simulink model "new_envModel_rl"  (R2020b)
settings: Solver=ode23t  StartTime=0.0  StopTime=8  RelTol=1e-2
values from neighbouring files (symbols this model uses):
  simlen = 80    [new_main_rl.m]    (also in old_main_rl.m = 5)
  Tf = simlen*Ts    [new_main_rl.m]    (also in old_main_rl.m)
  Ts = s.Ts    [new_main_rl.m]    (also in old_main_rl.m)
  ulim = s.actuatorRange    [new_main_rl.m]    (also in old_main_rl.m)
  whichAg_sim = whichAg_sim*5    (= 30)    [new_main_rl.m]    (also in old_main_rl.m)
  ylim = s.sensorRange    [new_main_rl.m]    (also in old_main_rl.m)
undefined symbols (not defined in the file or in its folder): s
libraries: rllib x3, simulink x2
settings Model: Creator=The MathWorks, Inc.  LastModifiedBy=sunan
settings DataIOCC: ExternalInput=s  SaveFormat=Structure  SaveOutput=off  SignalLogging=off  InspectSignalLogs=on  SaveTime=off  DSMLoggingName=s

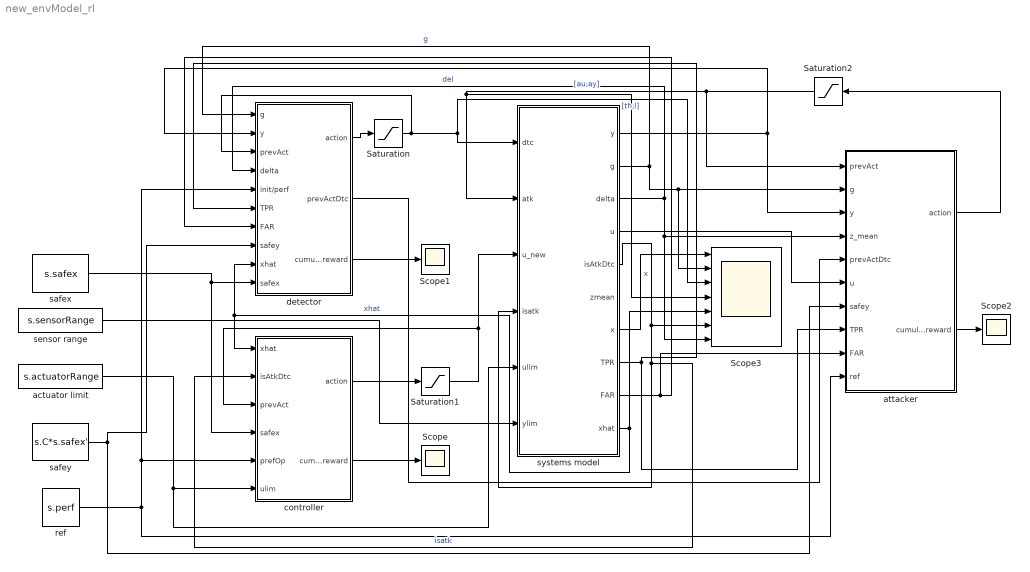
== system new_envModel_rl ==
  Saturation : Saturate  UpperLimit=[100;simlen]  LowerLimit=[0;1]
  Saturation1 : Saturate  UpperLimit=s.actuatorRange  LowerLimit=-s.actuatorRange
  Saturation2 : Saturate  UpperLimit=[ulim;ylim]  LowerLimit=-[ulim;ylim]
  Scope : Scope
  Scope1 : Scope
  Scope2 : Scope
  Scope3 : Scope  NumInputPorts=7
  actuator limit : Constant  Value=s.actuatorRange
  attacker : Subsystem
  controller : Subsystem
  detector : Subsystem
  ref : Constant  Value=s.perf
  safex : Constant  Value=s.safex
  safey : Constant  Value=s.C*s.safex'
  sensor range : Constant  Value=s.sensorRange
  systems model : Subsystem
  wires:
  systems model/1(y) -> detector/2(y), attacker/3(y)
  ref/1 -> controller/5(prefOp), detector/5(init/perf), attacker/10(ref)
  safey/1 -> attacker/7(safey), detector/8(safey)
  systems model/3(delta) -> Scope3/7, attacker/4(z_mean), detector/4(delta)  "del"
  systems model/2(g) -> detector/1(g), Scope3/2, attacker/2(g)  "g"
  sensor range/1 -> systems model/6(ylim)
  actuator limit/1 -> systems model/5(ulim), controller/6(ulim)
  Saturation/1 -> detector/3(prevAct), Scope3/3, systems model/1(dtc)  "[th;l]"
  Saturation1/1 -> systems model/3(u_new), controller/3(prevAct)
  Saturation2/1 -> attacker/1(prevAct), systems model/2(atk), Scope3/4  "[au;ay]"
  systems model/7(x) -> Scope3/1  "x"
  systems model/9(FAR) -> detector/7(FAR), attacker/9(FAR)
  systems model/8(TPR) -> attacker/8(TPR), detector/6(TPR)
  detector/1(action) -> Saturation/1
  detector/3(cumulative_reward) -> Scope1/1
  systems model/5(isAtkDtc) -> systems model/4(isatk), controller/2(isAtkDtc), Scope3/6  "isatk"
  controller/1(action) -> Saturation1/1
  controller/2(cumulative_reward) -> Scope/1
  detector/2(prevActDtc) -> attacker/5(prevActDtc)
  systems model/4(u) -> attacker/6(u)
  attacker/1(action) -> Saturation2/1
  attacker/2(cumulative_reward) -> Scope2/1
  systems model/10(xhat) -> Scope3/5, controller/1(xhat), detector/9(xhat)  "xhat"
  safex/1 -> detector/10(safex), controller/4(safex)

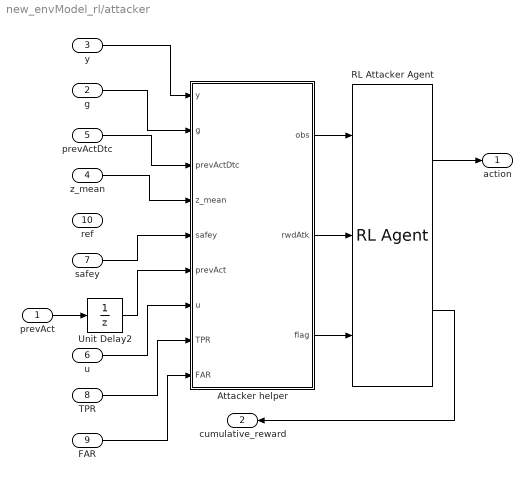
== system new_envModel_rl/attacker ==
  prevAct : Inport
  g : Inport  Port=2
  y : Inport  Port=3
  z_mean : Inport  Port=4
  prevActDtc : Inport  Port=5
  u : Inport  Port=6
  safey : Inport  Port=7
  TPR : Inport  Port=8
  FAR : Inport  Port=9
  ref : Inport  Port=10
  Attacker helper : Subsystem
  RL Attacker Agent : rllib/RL Agent  Agent=agentAtk  ProvideReward=on  ProvideIsDone=on  ProvideCumRwd=on  TreatAsDirectFeedthrough=on  CollectLoggedSignals=on  CollectModelStates=on
  Unit Delay2 : UnitDelay  SampleTime=-1  HasFrameUpgradeWarning=on
  action : Outport
  cumulative_reward : Outport  Port=2
  wires:
  z_mean/1 -> Attacker helper/4(z_mean)
  prevAct/1 -> Unit Delay2/1
  y/1 -> Attacker helper/1(y)
  Attacker helper/3(flag) -> RL Attacker Agent/3
  Attacker helper/1(obs) -> RL Attacker Agent/1
  Attacker helper/2(rwdAtk) -> RL Attacker Agent/2
  RL Attacker Agent/2 -> cumulative_reward/1
  Unit Delay2/1 -> Attacker helper/6(prevAct)
  RL Attacker Agent/1 -> action/1
  TPR/1 -> Attacker helper/8(TPR)
  FAR/1 -> Attacker helper/9(FAR)
  prevActDtc/1 -> Attacker helper/3(prevActDtc)
  g/1 -> Attacker helper/2(g)
  u/1 -> Attacker helper/7(u)
  safey/1 -> Attacker helper/5(safey)

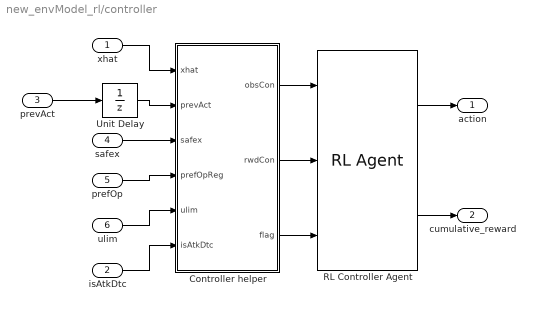
== system new_envModel_rl/controller ==
  xhat : Inport
  isAtkDtc : Inport  Port=2
  prevAct : Inport  Port=3
  safex : Inport  Port=4
  prefOp : Inport  Port=5
  ulim : Inport  Port=6
  Controller helper : Subsystem
  RL Controller Agent : rllib/RL Agent  Agent=agentCon  ProvideReward=on  ProvideIsDone=on  ProvideCumRwd=on  TreatAsDirectFeedthrough=on  CollectLoggedSignals=on  CollectModelStates=on
  Unit Delay : UnitDelay  SampleTime=-1  HasFrameUpgradeWarning=on
  action : Outport
  cumulative_reward : Outport  Port=2
  wires:
  Unit Delay/1 -> Controller helper/2(prevAct)
  RL Controller Agent/2 -> cumulative_reward/1
  prefOp/1 -> Controller helper/4(prefOpReg)
  Controller helper/1(obsCon) -> RL Controller Agent/1
  ulim/1 -> Controller helper/5(ulim)
  Controller helper/3(flag) -> RL Controller Agent/3
  safex/1 -> Controller helper/3(safex)
  prevAct/1 -> Unit Delay/1
  Controller helper/2(rwdCon) -> RL Controller Agent/2
  isAtkDtc/1 -> Controller helper/6(isAtkDtc)
  RL Controller Agent/1 -> action/1
  xhat/1 -> Controller helper/1(xhat)

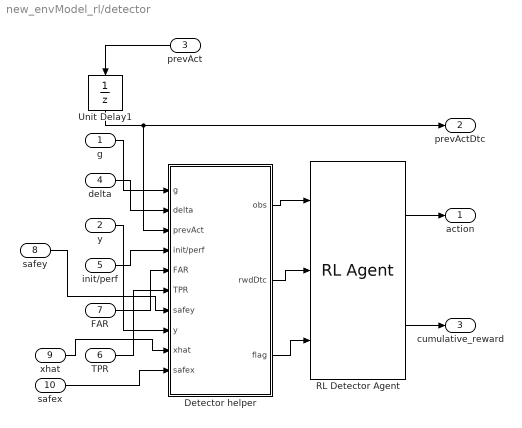
== system new_envModel_rl/detector ==
  g : Inport
  y : Inport  Port=2
  prevAct : Inport  Port=3
  delta : Inport  Port=4
  init/perf : Inport  Port=5
  TPR : Inport  Port=6
  FAR : Inport  Port=7
  safey : Inport  Port=8
  xhat : Inport  Port=9
  safex : Inport  Port=10
  Detector helper : Subsystem
  RL Detector Agent : rllib/RL Agent  Agent=agentDtc  ProvideReward=on  ProvideIsDone=on  ProvideCumRwd=on  TreatAsDirectFeedthrough=on  CollectLoggedSignals=on  CollectModelStates=on
  Unit Delay1 : UnitDelay  SampleTime=-1  HasFrameUpgradeWarning=on
  action : Outport
  prevActDtc : Outport  Port=2
  cumulative_reward : Outport  Port=3
  wires:
  FAR/1 -> Detector helper/5(FAR)
  TPR/1 -> Detector helper/6(TPR)
  g/1 -> Detector helper/1(g)
  prevAct/1 -> Unit Delay1/1
  RL Detector Agent/2 -> cumulative_reward/1
  Detector helper/3(flag) -> RL Detector Agent/3
  Detector helper/1(obs) -> RL Detector Agent/1
  Detector helper/2(rwdDtc) -> RL Detector Agent/2
  RL Detector Agent/1 -> action/1
  init/perf/1 -> Detector helper/4(init/perf)
  delta/1 -> Detector helper/2(delta)
  Unit Delay1/1 -> prevActDtc/1, Detector helper/3(prevAct)
  y/1 -> Detector helper/8(y)
  safey/1 -> Detector helper/7(safey)
  xhat/1 -> Detector helper/9(xhat)
  safex/1 -> Detector helper/10(safex)

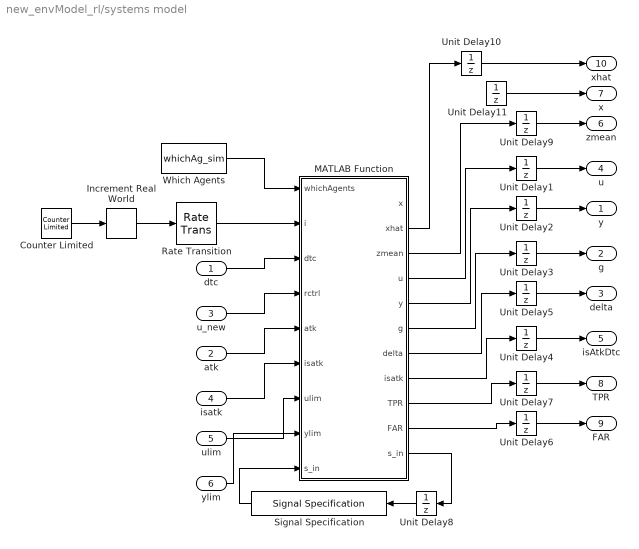
== system new_envModel_rl/systems model ==
  dtc : Inport
  atk : Inport  Port=2
  u_new : Inport  Port=3
  isatk : Inport  Port=4
  ulim : Inport  Port=5
  ylim : Inport  Port=6
  Counter Limited : simulink/Sources/Counter Limited  uplimit=Tf/Ts-2  tsamp=Ts
  Increment Real World : simulink/Additional Math & Discrete/Additional Math: Increment - Decrement/Increment Real World
      settings: SourceProductBaseCode=SL
  MATLAB Function : MATLAB Function  TreatAsAtomicUnit=on
  Rate Transition : RateTransition
  Signal Specification : SignalSpecification  OutDataTypeStr=Bus: slBus1  BusOutputAsStruct=on
  Unit Delay{1..7,9..11} (10 alike) : UnitDelay  SampleTime=-1  HasFrameUpgradeWarning=on
  Unit Delay8 : UnitDelay  InitialCondition=s  SampleTime=-1  HasFrameUpgradeWarning=on
  Which Agents : Constant  Value=whichAg_sim  SampleTime=Ts
  y : Outport
  g : Outport  Port=2
  delta : Outport  Port=3
  u : Outport  Port=4
  isAtkDtc : Outport  Port=5
  zmean : Outport  Port=6
  x : Outport  Port=7
  TPR : Outport  Port=8
  FAR : Outport  Port=9
  xhat : Outport  Port=10
  wires:
  Unit Delay9/1 -> zmean/1
  Unit Delay7/1 -> TPR/1
  Unit Delay6/1 -> FAR/1
  Unit Delay2/1 -> y/1
  MATLAB Function/9(TPR) -> Unit Delay7/1
  Unit Delay3/1 -> g/1
  Unit Delay4/1 -> isAtkDtc/1
  Unit Delay5/1 -> delta/1
  Increment Real World/1 -> Rate Transition/1
  Rate Transition/1 -> MATLAB Function/2(i)
  MATLAB Function/6(g) -> Unit Delay3/1
  MATLAB Function/7(delta) -> Unit Delay5/1
  ulim/1 -> MATLAB Function/7(ulim)
  Which Agents/1 -> MATLAB Function/1(whichAgents)
  MATLAB Function/5(y) -> Unit Delay2/1
  Unit Delay1/1 -> u/1
  isatk/1 -> MATLAB Function/6("isatk ")
  ylim/1 -> MATLAB Function/8(ylim)
  Counter Limited/1 -> Increment Real World/1
  MATLAB Function/4(u) -> Unit Delay1/1
  atk/1 -> MATLAB Function/5(atk)
  dtc/1 -> MATLAB Function/3(dtc)
  MATLAB Function/8(isatk) -> Unit Delay4/1
  u_new/1 -> MATLAB Function/4(rctrl)
  ? -> Unit Delay11/1
  MATLAB Function/3(zmean) -> Unit Delay9/1
  MATLAB Function/10(FAR) -> Unit Delay6/1
  MATLAB Function/11(s_in) -> Unit Delay8/1
  Signal Specification/1 -> MATLAB Function/9("s_in ")
  Unit Delay8/1 -> Signal Specification/1
  MATLAB Function/2(xhat) -> Unit Delay10/1
  Unit Delay11/1 -> x/1
  Unit Delay10/1 -> xhat/1

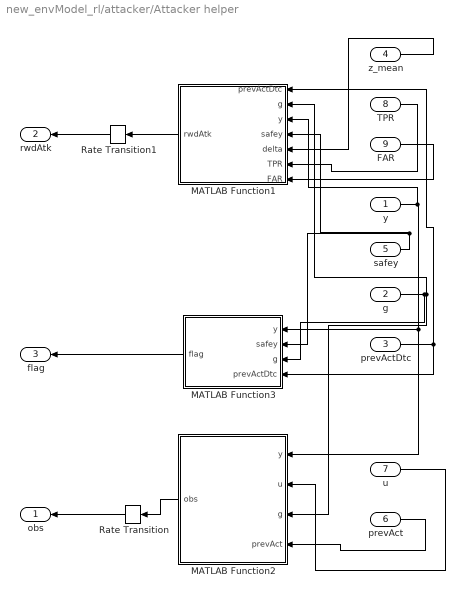
== system new_envModel_rl/attacker/Attacker helper ==
  y : Inport
  g : Inport  Port=2
  prevActDtc : Inport  Port=3
  z_mean : Inport  Port=4
  safey : Inport  Port=5
  prevAct : Inport  Port=6
  u : Inport  Port=7
  TPR : Inport  Port=8
  FAR : Inport  Port=9
  MATLAB Function1 : MATLAB Function  TreatAsAtomicUnit=on
  MATLAB Function2 : MATLAB Function  TreatAsAtomicUnit=on
  MATLAB Function3 : MATLAB Function  TreatAsAtomicUnit=on
  Rate Transition : RateTransition
  Rate Transition1 : RateTransition
  obs : Outport
  rwdAtk : Outport  Port=2
  flag : Outport  Port=3
  wires:
  MATLAB Function1/1(rwdAtk) -> Rate Transition1/1
  z_mean/1 -> MATLAB Function1/5(delta)
  prevAct/1 -> MATLAB Function2/4(prevAct)
  u/1 -> MATLAB Function2/2(u)
  TPR/1 -> MATLAB Function1/6(TPR)
  MATLAB Function3/1(flag) -> flag/1
  FAR/1 -> MATLAB Function1/7(FAR)
  Rate Transition/1 -> obs/1
  safey/1 -> MATLAB Function1/4(safey), MATLAB Function3/2(safey)
  MATLAB Function2/1(obs) -> Rate Transition/1
  Rate Transition1/1 -> rwdAtk/1
  prevActDtc/1 -> MATLAB Function3/4(prevActDtc), MATLAB Function1/1(prevActDtc)
  y/1 -> MATLAB Function2/1(y), MATLAB Function3/1(y), MATLAB Function1/3(y)
  g/1 -> MATLAB Function2/3(g), MATLAB Function1/2(g), MATLAB Function3/3(g)

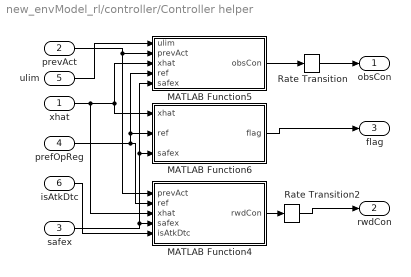
== system new_envModel_rl/controller/Controller helper ==
  xhat : Inport
  prevAct : Inport  Port=2
  safex : Inport  Port=3
  prefOpReg : Inport  Port=4
  ulim : Inport  Port=5
  isAtkDtc : Inport  Port=6
  MATLAB Function4 : MATLAB Function  TreatAsAtomicUnit=on
  MATLAB Function5 : MATLAB Function  TreatAsAtomicUnit=on
  MATLAB Function6 : MATLAB Function  TreatAsAtomicUnit=on
  Rate Transition : RateTransition
  Rate Transition2 : RateTransition
  obsCon : Outport
  rwdCon : Outport  Port=2
  flag : Outport  Port=3
  wires:
  prefOpReg/1 -> MATLAB Function6/2(ref), MATLAB Function5/4(ref), MATLAB Function4/2(ref)
  safex/1 -> MATLAB Function5/5(safex), MATLAB Function6/3(safex), MATLAB Function4/4(safex)
  MATLAB Function4/1(rwdCon) -> Rate Transition2/1
  MATLAB Function5/1(obsCon) -> Rate Transition/1
  xhat/1 -> MATLAB Function6/1(xhat), MATLAB Function5/3(xhat), MATLAB Function4/3(xhat)
  prevAct/1 -> MATLAB Function4/1(prevAct), MATLAB Function5/2(prevAct)
  Rate Transition/1 -> obsCon/1
  MATLAB Function6/1(flag) -> flag/1
  ulim/1 -> MATLAB Function5/1(ulim)
  Rate Transition2/1 -> rwdCon/1
  isAtkDtc/1 -> MATLAB Function4/5(isAtkDtc)

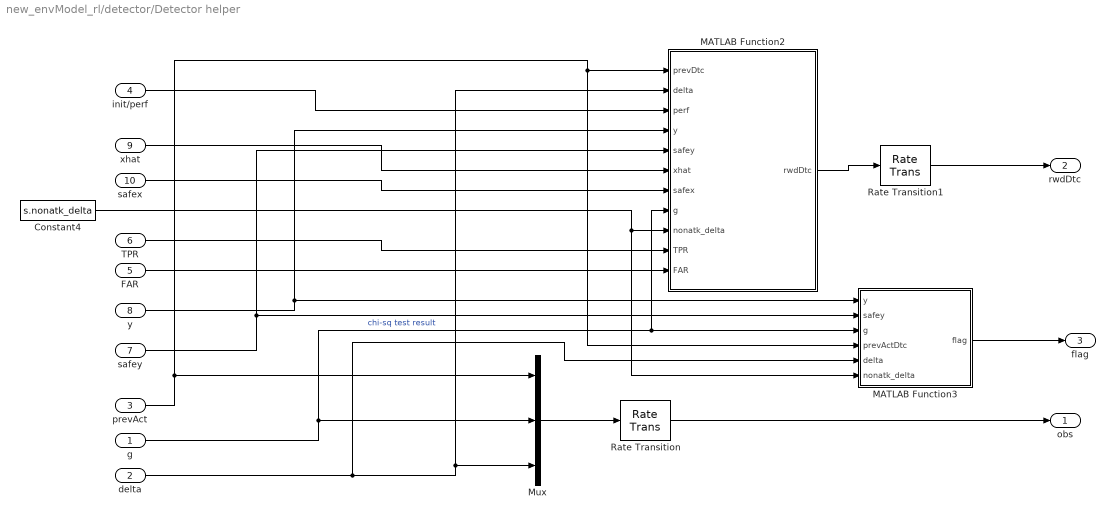
== system new_envModel_rl/detector/Detector helper ==
  g : Inport
  delta : Inport  Port=2
  prevAct : Inport  Port=3
  init/perf : Inport  Port=4
  FAR : Inport  Port=5
  TPR : Inport  Port=6
  safey : Inport  Port=7
  y : Inport  Port=8
  xhat : Inport  Port=9
  safex : Inport  Port=10
  Constant4 : Constant  Value=s.nonatk_delta  SampleTime=Ts
  MATLAB Function2 : MATLAB Function  TreatAsAtomicUnit=on
  MATLAB Function3 : MATLAB Function  TreatAsAtomicUnit=on
  Mux : Mux  Inputs=3
  Rate Transition : RateTransition
  Rate Transition1 : RateTransition
  obs : Outport
  rwdDtc : Outport  Port=2
  flag : Outport  Port=3
  wires:
  MATLAB Function3/1(flag) -> flag/1
  Rate Transition/1 -> obs/1
  prevAct/1 -> MATLAB Function2/1(prevDtc), MATLAB Function3/4(prevActDtc), Mux/1
  Mux/1 -> Rate Transition/1
  g/1 -> MATLAB Function2/8(g), MATLAB Function3/3(g), Mux/2  "chi-sq test result"
  delta/1 -> MATLAB Function3/5(delta), MATLAB Function2/2(delta), Mux/3
  init/perf/1 -> MATLAB Function2/3(perf)
  TPR/1 -> MATLAB Function2/10(TPR)
  Constant4/1 -> MATLAB Function2/9(nonatk_delta), MATLAB Function3/6(nonatk_delta)
  FAR/1 -> MATLAB Function2/11(FAR)
  y/1 -> MATLAB Function2/4(y), MATLAB Function3/1(y)
  safey/1 -> MATLAB Function2/5(safey), MATLAB Function3/2(safey)
  MATLAB Function2/1(rwdDtc) -> Rate Transition1/1
  Rate Transition1/1 -> rwdDtc/1
  xhat/1 -> MATLAB Function2/6(xhat)
  safex/1 -> MATLAB Function2/7(safex)

== matlab function new_envModel_rl/controller/Controller helper/MATLAB Function5 ==
  data: ulim input; obsCon output; prevAct input; xhat input; ref input; safex input
function obsCon = obsCon(ulim,prevAct,xhat,ref,safex)
   
    obsCon=[ulim;prevAct;xhat];

== matlab function new_envModel_rl/controller/Controller helper/MATLAB Function6 ==
  data: xhat input; ref input; flag output; safex input
function flag = stop(xhat,ref,safex)
% flag= 0;
state_max_in = max((-abs(xhat)+abs(ref))'); % to find this minimum inclusion
flag = min(state_max_in');

== matlab function new_envModel_rl/detector/Detector helper/MATLAB Function3 ==
  data: y input; flag output; safey input; g input; prevActDtc input; delta input; nonatk_delta input
function flag  = stop(y,safey, g, prevActDtc,delta,nonatk_delta)
%     format long g;
    th = abs(prevActDtc(1));
%     flag = g < th && ((delta > nonatk_delta) || (abs(y)> abs(safey)));
flag= 0;

== matlab function new_envModel_rl/detector/Detector helper/MATLAB Function2 ==
  data: prevDtc input; rwdDtc output; delta input; perf input; y input; safey input; xhat input; safex input; g input; nonatk_delta input; TPR input; FAR input
function rwdDtc   = rwdDtcCalc(prevDtc,delta,perf,y,safey,xhat,safex,g,nonatk_delta,TPR,FAR)
%    format long g;
    th = prevDtc(1);
    l = prevDtc(2);
    state_in_pref = max((abs(xhat)>abs(perf))'); % to check if estimated state lies within prefereble range
    state_max_out = min((abs(xhat)-abs(perf))'); % to find this maximum violation
    % if attacked i.e. non-centrality high, either of the estimated states
    % are outside
    if (delta > nonatk_delta) || max(state_in_pref')%max(abs(xhat)>abs(init.*safex))%(abs(y)> abs(safey))
        disp("under attack: increase tpr")
%         rwdDtc = 100*TPR*(TPR>=0.9)+ 100*(g>th)*(g-th)/th- 50*max(abs(y)-abs(safey))/max(abs(safey))
%         rwdDtc = 100*(g>th)+ 150*(g-th) + 100*(TPR-0.9)- 50*(th>g)*max(abs(y)-abs(safey))/max(abs(safey))
%         rwdDtc = 100*(g>th)+ 150*(g-th) + 100*(TPR-0.9)- 50*(th>g)*max(abs(xhat)-abs(init.*safex))/max(abs(init.*safex))
        rwdDtc = 100*(g>th)+ 150*(g-th) + 100*(TPR-0.9)- 50*(th>g)*min(state_max_out)/max(abs(perf(1,:)))
    else
        disp("no attack: reduce far")
        rwdDtc = 100*(1-FAR)*(FAR<0.05) + 100*(g<th)+150*(th-g)
    end
end

% removing th from denomenator..because th= 0 is possible nd th has no unit

== matlab function new_envModel_rl/attacker/Attacker helper/MATLAB Function1 ==
  data: rwdAtk output; prevActDtc input; g input; y input; safey input; delta input; TPR input; FAR input
function rwdAtk  = rwrdAtk(prevActDtc,g,y,safey,delta,TPR,FAR)
%    format long g;
   th = abs(prevActDtc(1));
   tau = max(1,ceil(prevActDtc(2,1)));
   dof = size(y,1)*(tau);
   op_unsafe = max((abs(y)>abs(safey'))'); % to check if the output is outside the preferebale range
   op_unsafety = max(abs(y)-abs(safey'));
%    FAR = chi2cdf(th,dof,'upper')
%    TPR = ncx2cdf(th,dof,abs(delta),'upper');
%    rwdAtk = FAR/TPR + 50*(g<th)+ 100*(y-ref)^2;
%             50*(FAR-0.05)-40*TPR + 50*(g<th)+ 100*(abs(y)-abs(safey))
% % rwdAtk = 50*(1-FAR) -50*TPR + 100*(g<th & abs(y)>abs(safey))+ 100*(abs(y)-abs(safey))
% rwdAtk = 50*(-FAR) -50*TPR + 100*(g<th)*(abs(y)-abs(safey))+ 100*(g<th)*(abs(y)-0.4*abs(safey))
% rwdAtk = 50*(FAR) -100*TPR + 100*max(abs(y)-abs(safey))/max(abs(safey))+250*(th-g)...
%     +100*(g<th & abs(y)>abs(safey))
    rwdAtk = 50*(FAR) -100*TPR + 100*max(op_unsafety')/min(abs(safey(:,1)'))+250*(th-g)...
    +100*(g<th & max(op_unsafe'))

% 50*(FAR) -100*TPR + 50*max(abs(y)...
%     -abs(safey))/max(abs(safey))+150*(th-g) +100*(abs(y)>abs(safey))*(g<=th)

%  50*(FAR) -100*TPR + 100*(g<=th)*max(abs(y)-abs(safey))/max(abs(safey))...
%                                 +100*(abs(y)>abs(safey))*(g<=th)*(th-g)/th
% removing th from denomenator..because th= 0 is possible nd th hsa no unit

== matlab function new_envModel_rl/systems model/MATLAB Function ==
  data: x output; xhat output; zmean output; whichAgents input; u output; i input; y output; g output; delta output; dtc input; rctrl input; atk input; isatk input; ulim input; ylim input; isatk output; TPR output; FAR output; s_in output; s_in input Bus: slBus1; atkOn parameter
function [x,xhat,zmean,u,y,g,delta,isatk,TPR,FAR,s_in] = env(whichAgents,i,dtc,rctrl,atk,isatk,ulim,ylim,s_in, atkOn)
% function [y,g,z_mean]= envSys(atk,dtc,new_u,ref, s)
%% SYS_ENV progress every iteration goes here
disp("-------------iteration: "+i+"--------------")
%% init vars
xdim= size(s_in.A,2);
ydim= size(s_in.C,1);
udim= size(s_in.B,2);
au= zeros(udim,1);
ay= zeros(ydim,1);
%% check which agents are activated, if attack is on for this episode
if ~rem(whichAgents,2)
    disp("with attacker agent");
    for i1=1:udim
        au(i1,1)= atk(i1,1)
    end
    for i2=1:udim
        ay(i2,1)= atk(udim+i2,1)
    end  
else
    disp("without attacker agent, no attack");
    au=zeros(udim,1);
    ay=zeros(ydim,1);
end
if ~atkOn
    disp(" no attack FAR test");
    au=zeros(udim,1);
    ay=zeros(ydim,1);
end
% 3 for controller agent
if ~rem(whichAgents,3)
    u_new= rctrl;
    disp("with controller agent");
else
    u_new = s_in.u_act(:,i);
    disp("without controller agent, with default control action");
end
% 5 for detector agent
if ~rem(whichAgents,5)
    th= abs(dtc(1))
    dtc_windw= max(1,(ceil(dtc(2))))
%     prevDtc = dtc;
    disp("with detector agent");
else
    disp("without detector agent, with default threshold, dof");
    th=s_in.th
    dtc_windw=1
%     prevDtc= [th;dtc_windw];
end

%% state progressions
          if isatk==0
%             s_in.t(i+1)=s_in.t(i)+s_in.Ts;

            s_in.a_u(:,i)=au.*s_in.uatkon;

            s_in.a_y(:,i)=ay.*s_in.yatkon;
          else
              
            s_in.a_u(:,i)=0;%au.*s_in.uatkon;

            s_in.a_y(:,i)=0;%ay.*s_in.yatkon;
          end
           
            s_in.est_err(:,i)= s_in.x_act(:,i)-s_in.xhat(:,i);
            
            s_in.u_act(:,i)= max(-ulim,min(ulim,s_in.K*s_in.xhat(:,i)));
            
            s_in.uatk(:,i)= max(-ulim,min(ulim,s_in.u_act(:,i)+s_in.a_u(:,i)));
            
            s_in.y_act(:,i)= max(-ylim,min(ylim,s_in.C*s_in.x_act(:,i))+s_in.meas_noise(:,i));
            
            s_in.yatk(:,i)= max(-ylim,min(ylim,s_in.y_act(:,i)+s_in.a_y(:,i)));
            
            s_in.z(:,i)= s_in.yatk(:,i)-s_in.C*s_in.xhat(:,i);
            
            s_in.x_act(:,i+1) = s_in.A*s_in.x_act(:,i)-s_in.B*s_in.uatk(:,i)+s_in.proc_noise(:,i);

            s_in.xhat(:,i+1) = s_in.A*s_in.xhat(:,i) - s_in.B*s_in.u_act(:,i) + s_in.L*s_in.z(:,i);
%             assignin('base','s_in.xhat', s_in.xhat);
 
%             disp("print check values");
%             a_u= s_in.a_u(:,end)
%             a_y= s_in.a_y(:,end)
%             xval= s_in.x_act
%             xhat= s_in.xhat
%             esterr= s_in.est_err
%             uval= s_in.u_act
%             uatk= s_in.uatk
%             yval= s_in.y_act
%             yatk= s_in.yatk
%             Cxhat= s_in.C*s_in.xhat
            
            for i3=1:size(s_in.z,1)
                disp("print: checking mean calc: z_mean,var")
                z_current=s_in.z(i3,1:i)';
                mean(z_current)'
                var(z_current)'
                s_in.z_mean(i3,i)= mean(z_current)';
                s_in.z_var(i3,i) = var(z_current)';
                
            end
            disp("print checking z_val");
%             zval= [s_in.z(1,1:i+1);s_in.z(2,1:i+1)]
            s_in.chi_tst(i)= (s_in.z(:,i)'/s_in.nonatk_zvar)*s_in.z(:,i); % ttc without noise z var=0.1
%             s_in.chi_tst(i+1)= s_in.z(:,i+1)'*inv(cov(s_in.z'))*s_in.z(:,i+1);
%              if ~isfinite(s_in.chi_tst(i))
%                     s_in.chi_tst(i)= 0;
%              end
            s_in.threshold(i)= th;
            s_in.tau(i)= dtc_windw;
            s_in.g(i) = 0;
            s_in.non_cent(:,i)= 0;
%             if i-tau+1 > 0                  % Calculate detector window starting index
%                 srt = i-tau+1;              % tau is the detector window length
%             else
%                 srt = 1;
%             end
            disp("print z_cov");
            z_covar = cov( s_in.z(:,1:i)')
%             if det(z_covar)==0
%                 s_in.z_var(:,i+1)=s_in.z_var(:,i);
%                 disp("singular")
%             end
%             disp("print here");
%% Chi square test and non centrality calculation
            for k = max(1,i-s_in.tau(i)+1):i
                s_in.g(i) = s_in.g(i) + s_in.chi_tst(k);  % Calculate gk (chi2 test)
                currentzmean= s_in.z_mean;
                disp("print checking non_cent");
                del= (s_in.z_mean(:,k)'/z_covar)*s_in.z_mean(:,k)
%                 del= s_in.z_mean(:,k+1)'*inv(cov(s_in.z'))*s_in.z_mean(:,k+1);
                if isnan(del)
                    disp("print adding zero non_cent if value is nan");
                    s_in.non_cent(i)= s_in.non_cent(i) + 0;
                elseif isinf(del)
                    disp("print adding high value non_cent if value is Inf");
                    s_in.non_cent(i)= s_in.non_cent(i) + 1234;
                else
                    s_in.non_cent(i)= s_in.non_cent(i) + del;
                    disp("print adding finite non_cent");
                end
            end
%             noncent= s_in.non_cent(:,i)
%             disp("print chisq test val");
%             chitest= s_in.chi_tst(:,i)
%             gvals= s_in.g(:,i)
            ay_act= s_in.a_y(:,i);
            au_act = s_in.a_u(:,i);
% %% check state region
%         safey = (s_in.C*s_in.safex')';
%         perfy = (s_in.C*s_in.perf')';
%         unsafe_y = max((abs(y)-abs(safey'))'); % to check if the output is outside the preferebale range
%    op_unsafety = max(abs(y)-abs(safey'));
            
            
%% to start the RL based controller
%             if (max(abs(s_in.yatk(i))>abs(s_in.C*s_in.safex'))) || (s_in.g(i) > s_in.threshold(i))
              if (s_in.g(i) > s_in.threshold(i))
                  disp("detected");
                  isatk=isatk+1;
%               elseif (abs(s_in.yatk(i))<abs(s_in.C*s_in.safex'))
              elseif max(abs(s_in.xhat(:,i))<=abs(s_in.safex'))
                isatk=0;
              end
%               if isatk>0
%                 s_in.u_act(:,i) = max(-ulim,min(ulim,u_new));
%                 s_in.uatk(:,i)= max(-ulim,min(ulim,s_in.u_act(:,i)));%+s_in.a_u(:,i)));
%                 s_in.yatk(:,i)= max(-ylim,min(ylim,s_in.y_act(:,i)));%+s_in.a_y(:,i)));
%                 s_in.x_act(:,i+1) = s_in.A*s_in.x_act(:,i)-s_in.B*s_in.uatk(:,i)+s_in.proc_noise(:,i);
%                 s_in.xhat(:,i+1) = s_in.A*s_in.xhat(:,i) - s_in.B*s_in.u_act(:,i) + s_in.L*s_in.z(:,i);
% 
%                 
%                 ay_act= 0;
%                 au_act = 0;
%                 disp("detected");
%                 disp("print  new u");
%                 newu= s_in.u_act(:,i)
%                 newuatk= s_in.uatk(:,i);
%               elseif (abs(s_in.yatk(i))<abs(s_in.C*s_in.safex'))
%                 isatk=0;
%               end
              
            

    th= s_in.threshold(i)
    window= s_in.tau(i)
    dof= s_in.tau(i)*size(s_in.C,1)
    TPR= ncx2cdf(s_in.threshold(i),dof,s_in.non_cent(i),'upper')
    FAR= chi2cdf(s_in.threshold(i),dof,'upper')
    s_in.avgtpr(i)= TPR;
    s_in.avgfar(i)= FAR;
    avgtpr= mean(s_in.avgtpr)
    avgfar= mean(s_in.avgfar)
    g= s_in.g(i)
    
%     y= zeros(ydim,1);
%     x=zeros(xdim,1);
%     xhat=zeros(xdim,1);
%     u=zeros(udim,1);
%     zmean= zeros(ydim,1);
    
    y= s_in.yatk(:,i)
    u= s_in.uatk(:,i);
    delta = s_in.non_cent(i)
    
%     if (ay == ylim || ay == -ylim)
%         ay_act = ay- s_in.y_act(:,i);
%     end
%     if (au == ulim || au == -ulim)
%         au_act= au- s_in.u_act(:,i);
%     end
    fdi = [ay_act;au_act]
    x = s_in.x_act(:,i)
    xhat = s_in.xhat(:,i)
    zmean= s_in.z_mean(:,i);
	isatk
end

== matlab function new_envModel_rl/attacker/Attacker helper/MATLAB Function2 ==
  data: obs output; y input; u input; g input; prevAct input
function obs = obsAtk(y,u,g,prevAct)
%     format long g;
    ay= prevAct(1,1);
    au= prevAct(2,1);
    obs= [y;u;g;prevAct];

== matlab function new_envModel_rl/attacker/Attacker helper/MATLAB Function3 ==
  data: y input; flag output; safey input; g input; prevActDtc input
function flag  = stop(y,safey, g, prevActDtc)
%     format long g;
    th = abs(prevActDtc(1));
%     flag = g > th;
flag= 0;

== matlab function new_envModel_rl/controller/Controller helper/MATLAB Function4 ==
  data: rwdCon output; prevAct input; ref input; xhat input; safex input; isAtkDtc input
function rwdCon  = rwrdCon(prevAct,ref,xhat,safex,isAtkDtc)
%     format long g;
    u=prevAct;
%     ay=atk(2);
    %% safer : 0.5* safey
%     rwdCon = 350*(abs((y-ref)/ref) <= 0.30)-20*(prevAct)^2-100*(abs(y) > safey)-50
% rwdCon = isAtkDtc*(-(y-ref*safey)'*1000*(y-ref*safey))%-20*u^2
% rwdCon = isAtkDtc*(abs(ref*safey)-abs(y))'*1000*(abs(ref*safey)-abs(y))
% rwdCon = isAtkDtc*1000*max(abs(ref*safey)-abs(y))/max(abs(ref*safey))
    state_in_pref = max((abs(xhat)>abs(ref))'); % to check if estimated state lies within prefereble range
    state_max_in = max((-abs(xhat)+abs(ref))'); % to find this minimum inclusion
    rwdCon = isAtkDtc*1000*min(state_max_in)/min(abs(ref(1,:)))
